simulink model "flightControllerAltitude"  (R2016b)
settings: Solver=ode3  StartTime=0  StopTime=10.0  FixedStep=Ts  RelTol=1e-3  EnableMultiTasking=on
undefined symbols (not defined in the file): altitudeHoldValue, Controller
libraries: simulink x3
settings Model: Creator=The MathWorks, Inc.  LastModifiedBy=The MathWorks, Inc.
settings DataIOCC: LimitDataPoints=on  SaveFormat=Array
settings OptimizationCC: BlockReduction=off  DefaultParameterBehavior=Inlined  BufferReuse=off  LifeSpan=inf
settings DebuggingCC: AlgebraicLoopMsg=none  UnderspecifiedInitializationDetection=Classic  MergeDetectMultiDrivingBlocksExec=none  UnconnectedInputMsg=none  UnconnectedOutputMsg=none  UnconnectedLineMsg=none  AllowSymbolicDim=off  SFUnexpectedBacktrackingDiag=warning  SFNoUnconditionalDefaultTransitionDiag=warning  SFExecutionAtInitializationDiag=none
settings HardwareCC: ProdBitPerPointer=32  ProdBitPerSizeT=32  ProdBitPerPtrDiffT=32  ProdLargestAtomicFloat=None  ProdIntDivRoundTo=Undefined  ProdEndianess=Unspecified  ProdWordSize=32  ProdHWDeviceType=32-bit Generic
settings ModelReferenceCC: PropagateSignalLabelsOutOfModel=off
settings GRTTargetCC: TargetLangStandard=C89/C90 (ANSI)  GeneratePreprocessorConditionals=Disable all
settings ConfigComp: CovMetricSettings=dw  CovHtmlReporting=on  CovSaveCumulativeToWorkspaceVar=on  CovSaveSingleToWorkspaceVar=on  CovExternalEMLEnable=off  CovSFcnEnable=off

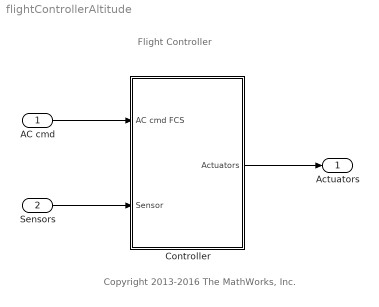
== system flightControllerAltitude ==
  note: Copyright 2013-2016 The MathWorks, Inc.
  note: Flight Controller
  AC cmd : Inport  OutDataTypeStr=Bus: CommandBus
  Sensors : Inport  Port=2  OutDataTypeStr=Bus: SensorsBus  BusOutputAsStruct=on
  Controller : Subsystem
      mask init:
      | controllerVars;
  Actuators : Outport
  wires:
  AC cmd/1 -> Controller/1(AC cmd FCS)
  Sensors/1 -> Controller/2(Sensor)
  Controller/1(Actuators) -> Actuators/1

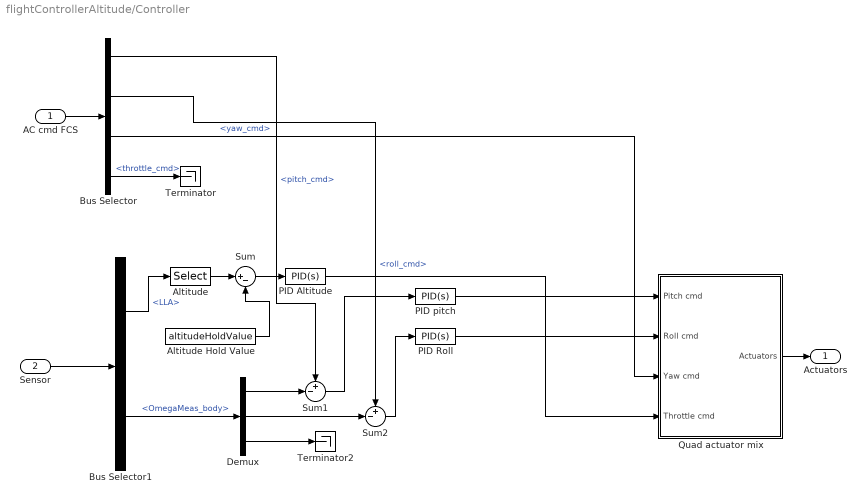
== system flightControllerAltitude/Controller ==
  AC cmd FCS : Inport
  Sensor : Inport  Port=2
  Altitude : Selector  InputPortWidth=3  IndexOptions=Index vector (dialog)  Indices=[3]  OutputSizes=1
  Altitude Hold Value : Constant  Value=altitudeHoldValue
  Bus Selector : BusSelector  OutputSignals=pitch_cmd,roll_cmd,yaw_cmd,throttle_cmd
  Bus Selector1 : BusSelector  OutputSignals=LLA,OmegaMeas_body
  Demux : Demux  Outputs=3
  PID Altitude : simulink/Continuous/PID Controller  Controller=PID  TimeDomain=Continuous-time  SampleTime=-1  IntegratorMethod=Forward Euler  FilterMethod=Forward Euler  Form=Parallel  UseFilter=on  ControllerParametersSource=internal  P=-114.050466183378  I=-0.999560878115567  D=-2891.38451636519  N=171.684827700763  InitialConditionSource=internal  InitialConditionForIntegrator=0  InitialConditionForFilter=0  ExternalReset=none  LimitOutput=off  UpperSaturationLimit=inf  LowerSaturationLimit=-inf  LinearizeAsGain=on  AntiWindupMode=none  Kb=1  TrackingMode=off  Kt=1  PParamMin=[]  PParamMax=[]  IParamMin=[]  IParamMax=[]  DParamMin=[]  DParamMax=[]  NParamMin=[]  NParamMax=[]  KbParamMin=[]  KbParamMax=[]  KtParamMin=[]  KtParamMax=[]  POutMin=[]  POutMax=[]  IOutMin=[]  IOutMax=[]  DOutMin=[]  DOutMax=[]  NOutMin=[]  NOutMax=[]  KbOutMin=[]  KbOutMax=[]  KtOutMin=[]  KtOutMax=[]  IntegratorOutMin=[]  IntegratorOutMax=[]  FilterOutMin=[]  FilterOutMax=[]  SumOutMin=[]  SumOutMax=[]  SumI1OutMin=[]  SumI1OutMax=[]  SumI2OutMin=[]  SumI2OutMax=[]  SumI3OutMin=[]  SumI3OutMax=[]  SumDOutMin=[]  SumDOutMax=[]  SaturationOutMin=[]  SaturationOutMax=[]  IntegratorContinuousStateAttributes=''  IntegratorStateMustResolveToSignalObject=off  IntegratorRTWStateStorageClass=Auto  FilterContinuousStateAttributes=''  FilterStateMustResolveToSignalObject=off  FilterRTWStateStorageClass=Auto  DifferentiatorICPrevScaledInput=0  DifferentiatorOutMin=[]  DifferentiatorOutMax=[]
  PID Roll : simulink/Continuous/PID Controller  Controller=PID  TimeDomain=Continuous-time  SampleTime=-1  IntegratorMethod=Forward Euler  FilterMethod=Forward Euler  Form=Parallel  UseFilter=on  ControllerParametersSource=internal  P=0.000785869263148391  I=0.000621245528289962  D=0.00024297273150912  N=155.924967958506  InitialConditionSource=internal  InitialConditionForIntegrator=0  InitialConditionForFilter=0  ExternalReset=none  LimitOutput=off  UpperSaturationLimit=inf  LowerSaturationLimit=-inf  LinearizeAsGain=on  AntiWindupMode=none  Kb=1  TrackingMode=off  Kt=1  PParamMin=[]  PParamMax=[]  IParamMin=[]  IParamMax=[]  DParamMin=[]  DParamMax=[]  NParamMin=[]  NParamMax=[]  KbParamMin=[]  KbParamMax=[]  KtParamMin=[]  KtParamMax=[]  POutMin=[]  POutMax=[]  IOutMin=[]  IOutMax=[]  DOutMin=[]  DOutMax=[]  NOutMin=[]  NOutMax=[]  KbOutMin=[]  KbOutMax=[]  KtOutMin=[]  KtOutMax=[]  IntegratorOutMin=[]  IntegratorOutMax=[]  FilterOutMin=[]  FilterOutMax=[]  SumOutMin=[]  SumOutMax=[]  SumI1OutMin=[]  SumI1OutMax=[]  SumI2OutMin=[]  SumI2OutMax=[]  SumI3OutMin=[]  SumI3OutMax=[]  SumDOutMin=[]  SumDOutMax=[]  SaturationOutMin=[]  SaturationOutMax=[]  IntegratorContinuousStateAttributes=''  IntegratorStateMustResolveToSignalObject=off  IntegratorRTWStateStorageClass=Auto  FilterContinuousStateAttributes=''  FilterStateMustResolveToSignalObject=off  FilterRTWStateStorageClass=Auto  DifferentiatorICPrevScaledInput=0  DifferentiatorOutMin=[]  DifferentiatorOutMax=[]
  PID pitch : simulink/Continuous/PID Controller  Controller=PID  TimeDomain=Continuous-time  SampleTime=-1  IntegratorMethod=Forward Euler  FilterMethod=Forward Euler  Form=Parallel  UseFilter=on  ControllerParametersSource=internal  P=-449.652681173872  I=-146.118873160313  D=-52.8378413871279  N=8.8075624027162  InitialConditionSource=internal  InitialConditionForIntegrator=0  InitialConditionForFilter=0  ExternalReset=none  LimitOutput=off  UpperSaturationLimit=inf  LowerSaturationLimit=-inf  LinearizeAsGain=on  AntiWindupMode=none  Kb=1  TrackingMode=off  Kt=1  PParamMin=[]  PParamMax=[]  IParamMin=[]  IParamMax=[]  DParamMin=[]  DParamMax=[]  NParamMin=[]  NParamMax=[]  KbParamMin=[]  KbParamMax=[]  KtParamMin=[]  KtParamMax=[]  POutMin=[]  POutMax=[]  IOutMin=[]  IOutMax=[]  DOutMin=[]  DOutMax=[]  NOutMin=[]  NOutMax=[]  KbOutMin=[]  KbOutMax=[]  KtOutMin=[]  KtOutMax=[]  IntegratorOutMin=[]  IntegratorOutMax=[]  FilterOutMin=[]  FilterOutMax=[]  SumOutMin=[]  SumOutMax=[]  SumI1OutMin=[]  SumI1OutMax=[]  SumI2OutMin=[]  SumI2OutMax=[]  SumI3OutMin=[]  SumI3OutMax=[]  SumDOutMin=[]  SumDOutMax=[]  SaturationOutMin=[]  SaturationOutMax=[]  IntegratorContinuousStateAttributes=''  IntegratorStateMustResolveToSignalObject=off  IntegratorRTWStateStorageClass=Auto  FilterContinuousStateAttributes=''  FilterStateMustResolveToSignalObject=off  FilterRTWStateStorageClass=Auto  DifferentiatorICPrevScaledInput=0  DifferentiatorOutMin=[]  DifferentiatorOutMax=[]
  Quad actuator mix : Subsystem
  Sum : Sum  Inputs=|+-
  Sum1 : Sum  Inputs=+-|
  Sum2 : Sum  Inputs=+-|
  Terminator : Terminator
  Terminator2 : Terminator
  Actuators : Outport
  wires:
  Quad actuator mix/1(Actuators) -> Actuators/1
  AC cmd FCS/1 -> Bus Selector/1
  Bus Selector/1 -> Sum1/1  "<pitch_cmd>"
  Bus Selector/2 -> Sum2/1  "<roll_cmd>"
  Bus Selector/3 -> Quad actuator mix/3(Yaw cmd)  "<yaw_cmd>"
  Bus Selector/4 -> Terminator/1  "<throttle_cmd>"
  Sensor/1 -> Bus Selector1/1
  Altitude Hold Value/1 -> Sum/2
  Bus Selector1/1 -> Altitude/1  "<LLA>"
  Altitude/1 -> Sum/1
  Sum/1 -> PID Altitude/1
  PID Altitude/1 -> Quad actuator mix/4(Throttle cmd)
  Bus Selector1/2 -> Demux/1  "<OmegaMeas_body>"
  Demux/1 -> Sum1/2
  Sum1/1 -> PID pitch/1
  Demux/2 -> Sum2/2
  Demux/3 -> Terminator2/1
  Sum2/1 -> PID Roll/1
  PID Roll/1 -> Quad actuator mix/2(Roll cmd)
  PID pitch/1 -> Quad actuator mix/1(Pitch cmd)

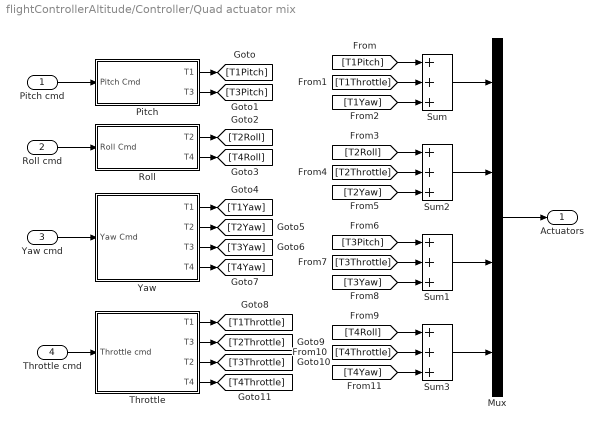
== system flightControllerAltitude/Controller/Quad actuator mix ==
  Pitch cmd : Inport
  Roll cmd : Inport  Port=2
  Yaw cmd : Inport  Port=3
  Throttle cmd : Inport  Port=4
  Mux : Mux
  Pitch : Subsystem
  Roll : Subsystem
  Sum{,1..3} (4 alike) : Sum  Inputs=+++
  Throttle : Subsystem
  Yaw : Subsystem
  Actuators : Outport
  wires:
  [T4Yaw] -> Sum3/3
  [T4Throttle] -> Sum3/2
  [T4Roll] -> Sum3/1
  [T3Yaw] -> Sum1/3
  [T3Throttle] -> Sum1/2
  [T3Pitch] -> Sum1/1
  Sum2/1 -> Mux/2
  [T2Yaw] -> Sum2/3
  [T2Throttle] -> Sum2/2
  [T2Roll] -> Sum2/1
  [T1Yaw] -> Sum/3
  [T1Throttle] -> Sum/2
  [T1Pitch] -> Sum/1
  Throttle/4(T4) -> [T4Throttle]
  Throttle/3(T2) -> [T3Throttle]
  Throttle/2(T3) -> [T2Throttle]
  Throttle/1(T1) -> [T1Throttle]
  Yaw/4(T4) -> [T4Yaw]
  Yaw/1(T1) -> [T1Yaw]
  Roll/2(T4) -> [T4Roll]
  Roll/1(T2) -> [T2Roll]
  Pitch/2(T3) -> [T3Pitch]
  Pitch/1(T1) -> [T1Pitch]
  Mux/1 -> Actuators/1
  Pitch cmd/1 -> Pitch/1(Pitch Cmd)
  Roll cmd/1 -> Roll/1(Roll Cmd)
  Yaw cmd/1 -> Yaw/1(Yaw Cmd)
  Throttle cmd/1 -> Throttle/1(Throttle cmd)
  Sum1/1 -> Mux/3
  Sum3/1 -> Mux/4
  Sum/1 -> Mux/1
  Yaw/2(T2) -> [T2Yaw]
  Yaw/3(T3) -> [T3Yaw]

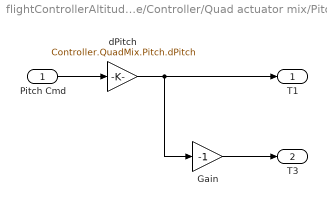
== system flightControllerAltitude/Controller/Quad actuator mix/Pitch ==
  Pitch Cmd : Inport
  Gain : Gain  Gain=-1
  dPitch : Gain  Gain=Controller.QuadMix.Pitch.dPitch
  T1 : Outport
  T3 : Outport  Port=2
  wires:
  Pitch Cmd/1 -> dPitch/1
  Gain/1 -> T3/1
  dPitch/1 -> T1/1, Gain/1

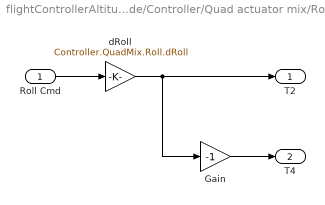
== system flightControllerAltitude/Controller/Quad actuator mix/Roll ==
  Roll Cmd : Inport
  Gain : Gain  Gain=-1
  dRoll : Gain  Gain=Controller.QuadMix.Roll.dRoll
  T2 : Outport
  T4 : Outport  Port=2
  wires:
  Gain/1 -> T4/1
  dRoll/1 -> Gain/1, T2/1
  Roll Cmd/1 -> dRoll/1

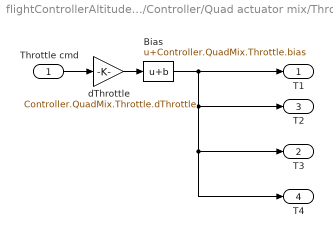
== system flightControllerAltitude/Controller/Quad actuator mix/Throttle ==
  Throttle cmd : Inport
  Bias : Bias  Bias=Controller.QuadMix.Throttle.bias
  dThrottle : Gain  Gain=Controller.QuadMix.Throttle.dThrottle
  T1 : Outport
  T3 : Outport  Port=2
  T2 : Outport  Port=3
  T4 : Outport  Port=4
  wires:
  Bias/1 -> T1/1, T2/1, T3/1, T4/1
  Throttle cmd/1 -> dThrottle/1
  dThrottle/1 -> Bias/1

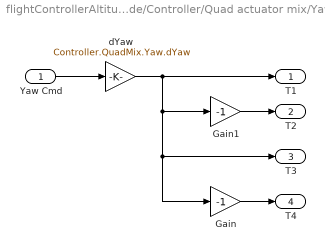
== system flightControllerAltitude/Controller/Quad actuator mix/Yaw ==
  Yaw Cmd : Inport
  Gain : Gain  Gain=-1
  Gain1 : Gain  Gain=-1
  dYaw : Gain  Gain=Controller.QuadMix.Yaw.dYaw
  T1 : Outport
  T2 : Outport  Port=2
  T3 : Outport  Port=3
  T4 : Outport  Port=4
  wires:
  Yaw Cmd/1 -> dYaw/1
  dYaw/1 -> T1/1, Gain1/1, T3/1, Gain/1
  Gain1/1 -> T2/1
  Gain/1 -> T4/1
